simulink model "delta"  (R2015b)
settings: Solver=VariableStepAuto  StartTime=0.0  StopTime=10.0  RelTol=1e-3
settings Model: Creator=yuji  LastModifiedBy=yuji

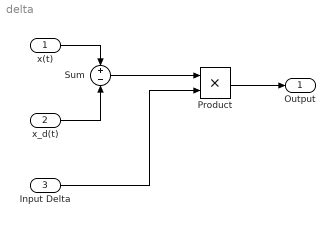
== system delta ==
  x(t) : Inport
  x_d(t) : Inport  Port=2
  Input Delta : Inport  Port=3
  Product : Product
  Sum : Sum  Inputs=+|-
  "Output " : Outport
  wires:
  x(t)/1 -> Sum/1
  x_d(t)/1 -> Sum/2
  Sum/1 -> Product/1
  Product/1 -> "Output "/1
  Input Delta/1 -> Product/2
